simulink model "Respuesta_Frenos"  (R2020a)
settings: Solver=VariableStepAuto  StartTime=0.0  StopTime=10  RelTol=1e-3
settings Model: Creator=Alejo  LastModifiedBy=USUARIO
settings DataIOCC: ReturnWorkspaceOutputs=off
settings DebuggingCC: ArithmeticOperatorsInVariantConditions=warning
settings SFSimCC: CustomCodeUndefinedFunction=UseInterfaceOnly

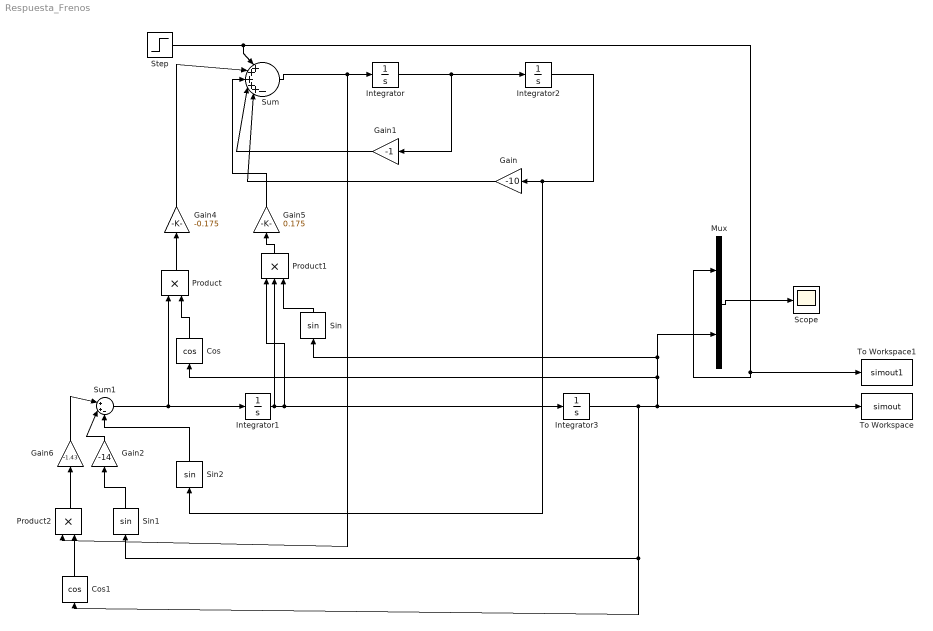
== system Respuesta_Frenos ==
  Cos : Trigonometry  Operator=cos
  Cos1 : Trigonometry  Operator=cos
  Gain : Gain  Gain=-10
  Gain1 : Gain  Gain=-1
  Gain2 : Gain  Gain=-14
  Gain4 : Gain  Gain=-0.175
  Gain5 : Gain  Gain=0.175
  Gain6 : Gain  Gain=-1.43
  Integrator{,1..3} (4 alike) : Integrator
  Mux : Mux  Inputs=2
  Product : Product
  Product1 : Product  Inputs=3
  Product2 : Product
  Scope : Scope
  Sin : Trigonometry
  Sin1 : Trigonometry
  Sin2 : Trigonometry
  Step : Step  Before=1  After=0  SampleTime=0.001
  Sum : Sum  Inputs=|+++++-
  Sum1 : Sum  Inputs=|++-
  To Workspace : ToWorkspace  VariableName=simout  SampleTime=-1
  To Workspace1 : ToWorkspace  VariableName=simout1  SampleTime=-1
  wires:
  Integrator1/1 -> Integrator3/1, Product1/1, Product1/2
  Integrator/1 -> Gain1/1, Integrator2/1
  Integrator2/1 -> Sin2/1, Gain/1
  Integrator3/1 -> Sin1/1, Cos1/1, To Workspace/1, Cos/1, Sin/1, Mux/2
  Sum1/1 -> Product/1, Integrator1/1
  Cos/1 -> Product/2
  Product/1 -> Gain4/1
  Sin/1 -> Product1/3
  Product1/1 -> Gain5/1
  Gain1/1 -> Sum/4
  Sum/1 -> Product2/1, Integrator/1
  Gain5/1 -> Sum/3
  Gain4/1 -> Sum/2
  Step/1 -> Mux/1, To Workspace1/1, Sum/1
  Mux/1 -> Scope/1
  Cos1/1 -> Product2/2
  Product2/1 -> Gain6/1
  Gain6/1 -> Sum1/1
  Sin1/1 -> Gain2/1
  Gain2/1 -> Sum1/2
  Gain/1 -> Sum/5
  Sin2/1 -> Sum1/3
